simulink model "headway_sim"  (R2020a)
settings: Solver=VariableStepAuto  StartTime=0.0  StopTime=800  RelTol=1e-3
values from neighbouring files (symbols this model uses):
  A = eval(A)    [headway.m]
  B = eval(B)    [headway.m]
  Cd = 1.2    [headway.m]
  i_e = 100    [headway.m]
  id1_ref = 0    [headway.m]
  id2_ref = 0    [headway.m]
  iq1_ref = (Fx1_ref)/((3/2)*(pi/tau)*(Ld*(M/Ld)*i_e))    (= 482.136730936)    [headway.m]
  iq2_ref = (Fx2_ref)/((3/2)*(pi/tau)*(Ld*(M/Ld)*i_e))    (= 482.136730936)    [headway.m]
  Ld = 0.06    [headway.m]
  Lq = 0.06    [headway.m]
  M = 0.1    [headway.m]
  m = 60000    [headway.m]
  p = 3    [headway.m]
  R = 1.04    [headway.m]
  rho = 1.225    [headway.m]
  Sa = 13    [headway.m]
  tau = 1    [headway.m]
  Vref = [Vq1_ref;Vd1_ref;Vq2_ref;Vd2_ref]    [headway.m]
  x_ref = [iq1_ref; id1_ref; iq2_ref; id2_ref; xdot_ref]    [headway.m]
undefined symbols (not defined in the file or in its folder): K
settings Model: Creator=adelina  LastModifiedBy=Federico

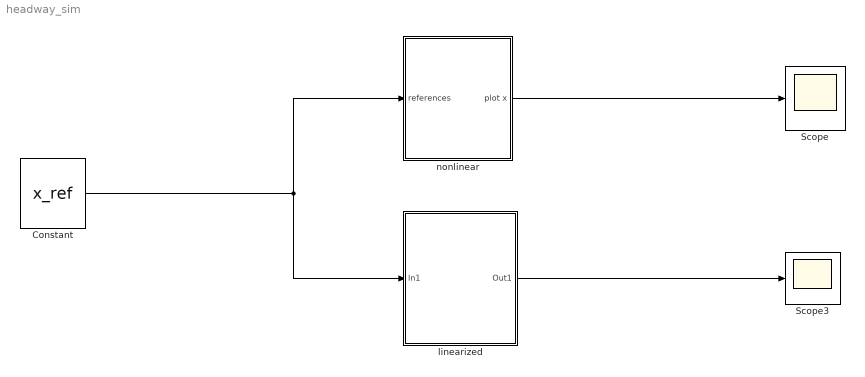
== system headway_sim ==
  Constant : Constant  Value=x_ref
  Scope : Scope
  Scope3 : Scope
  linearized : Subsystem
  nonlinear : Subsystem
  wires:
  Constant/1 -> nonlinear/1(references), linearized/1(In1)
  linearized/1(Out1) -> Scope3/1
  nonlinear/1(plot x) -> Scope/1

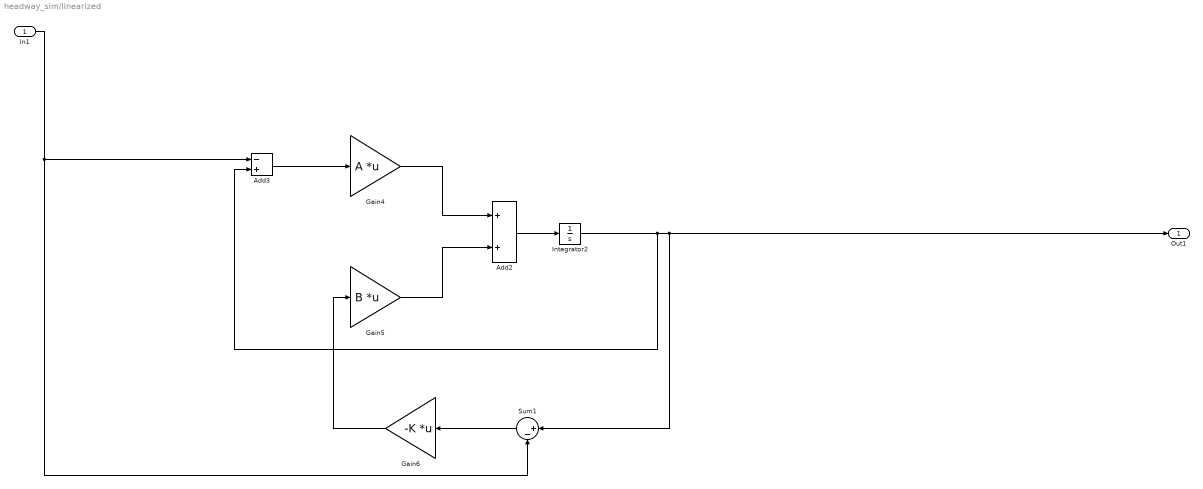
== system headway_sim/linearized ==
  In1 : Inport
  Add2 : Sum
  Add3 : Sum  Inputs=-+
  Gain4 : Gain  Gain=A  Multiplication=Matrix(K*u)
  Gain5 : Gain  Gain=B  Multiplication=Matrix(K*u)
  Gain6 : Gain  Gain=-K  Multiplication=Matrix(K*u)
  Integrator2 : Integrator  InitialCondition=[0;0;0;0;0]
  Sum1 : Sum  Inputs=|+-
  Out1 : Outport
  wires:
  Add2/1 -> Integrator2/1
  Gain5/1 -> Add2/2
  Gain6/1 -> Gain5/1
  Gain4/1 -> Add2/1
  Integrator2/1 -> Out1/1, Sum1/1, Add3/2
  Add3/1 -> Gain4/1
  In1/1 -> Sum1/2, Add3/1
  Sum1/1 -> Gain6/1

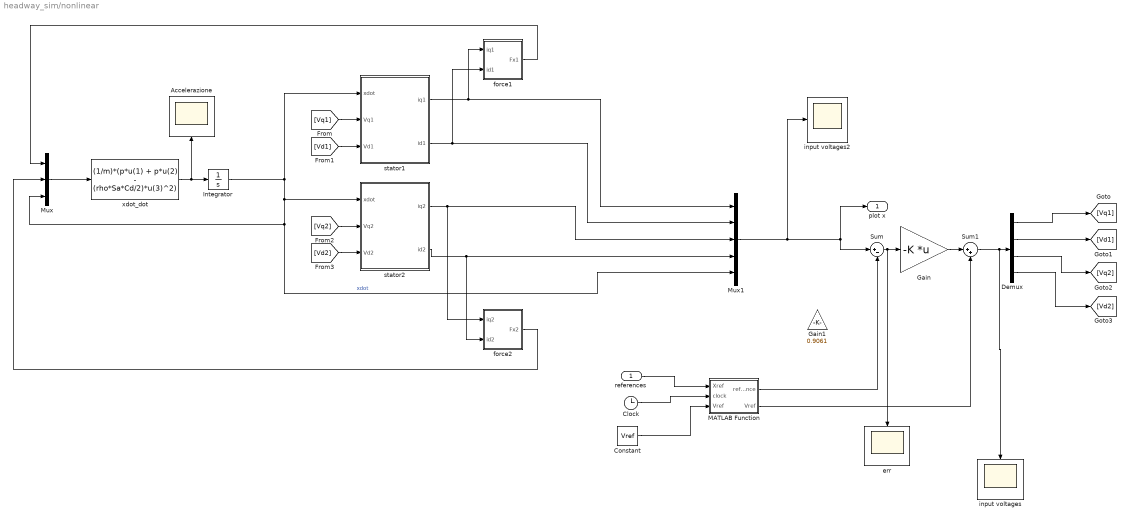
== system headway_sim/nonlinear ==
  references : Inport
  Accelerazione : Scope
  Clock : Clock
  Constant : Constant  Value=Vref
  Demux : Demux
  Gain : Gain  Gain=-K  Multiplication=Matrix(K*u)
  Gain1 : Gain  Gain=0.9061
  Integrator : Integrator
  MATLAB Function : MATLAB Function  TreatAsAtomicUnit=on
  Mux : Mux  Inputs=3
  Mux1 : Mux  Inputs=5
  Sum : Sum  Inputs=|+-
  Sum1 : Sum  Inputs=|++
  err : Scope
  force1 : Subsystem
  force2 : Subsystem
  input voltages : Scope
  input voltages2 : Scope
  stator1 : Subsystem
  stator2 : Subsystem
  xdot_dot : Fcn  Expr=(1/m)*(p*u(1) + p*u(2) - (rho*Sa*Cd/2)*u(3)^2)
  plot x : Outport
  wires:
  stator1/2(id1) -> Mux1/2, force1/2(id1)
  Mux1/1 -> input voltages2/1, Sum/1, plot x/1
  force1/1(Fx1) -> Mux/1
  Integrator/1 -> Mux/3, Mux1/5, stator2/1(xdot), stator1/1(xdot)  "xdot"
  Sum/1 -> Gain/1, err/1
  force2/1(Fx2) -> Mux/2
  stator2/1(iq2) -> force2/1("iq2 "), Mux1/3
  Mux/1 -> xdot_dot/1
  xdot_dot/1 -> Integrator/1, Accelerazione/1
  stator1/1(iq1) -> Mux1/1, force1/1("iq1 ")
  Demux/1 -> [Vq1]
  Demux/2 -> [Vd1]
  Demux/3 -> [Vq2]
  Demux/4 -> [Vd2]
  [Vq1] -> stator1/2(Vq1)
  [Vd1] -> stator1/3(Vd1)
  [Vq2] -> stator2/2(Vq2)
  [Vd2] -> stator2/3(Vd2)
  stator2/2(id2) -> force2/2(id2), Mux1/4
  Clock/1 -> MATLAB Function/2(clock)
  references/1 -> MATLAB Function/1(Xref)
  MATLAB Function/1(reference) -> Sum/2
  Gain/1 -> Sum1/1
  Sum1/1 -> input voltages/1, Demux/1
  MATLAB Function/2(Vref) -> Sum1/2
  Constant/1 -> MATLAB Function/3("Vref ")

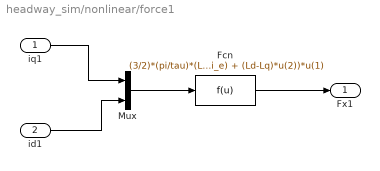
== system headway_sim/nonlinear/force1 ==
  "iq1 " : Inport
  id1 : Inport  Port=2
  Fcn : Fcn  Expr=(3/2)*(pi/tau)*(Ld*((M/Ld)*i_e) + (Ld-Lq)*u(2))*u(1)
  Mux : Mux  Inputs=2
  Fx1 : Outport
  wires:
  Fcn/1 -> Fx1/1
  "iq1 "/1 -> Mux/1
  id1/1 -> Mux/2
  Mux/1 -> Fcn/1

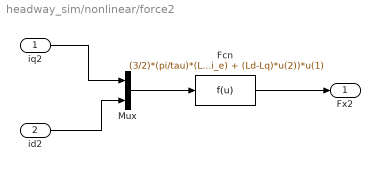
== system headway_sim/nonlinear/force2 ==
  "iq2 " : Inport
  id2 : Inport  Port=2
  Fcn : Fcn  Expr=(3/2)*(pi/tau)*(Ld*((M/Ld)*i_e) + (Ld-Lq)*u(2))*u(1)
  Mux : Mux  Inputs=2
  Fx2 : Outport
  wires:
  Fcn/1 -> Fx2/1
  "iq2 "/1 -> Mux/1
  id2/1 -> Mux/2
  Mux/1 -> Fcn/1

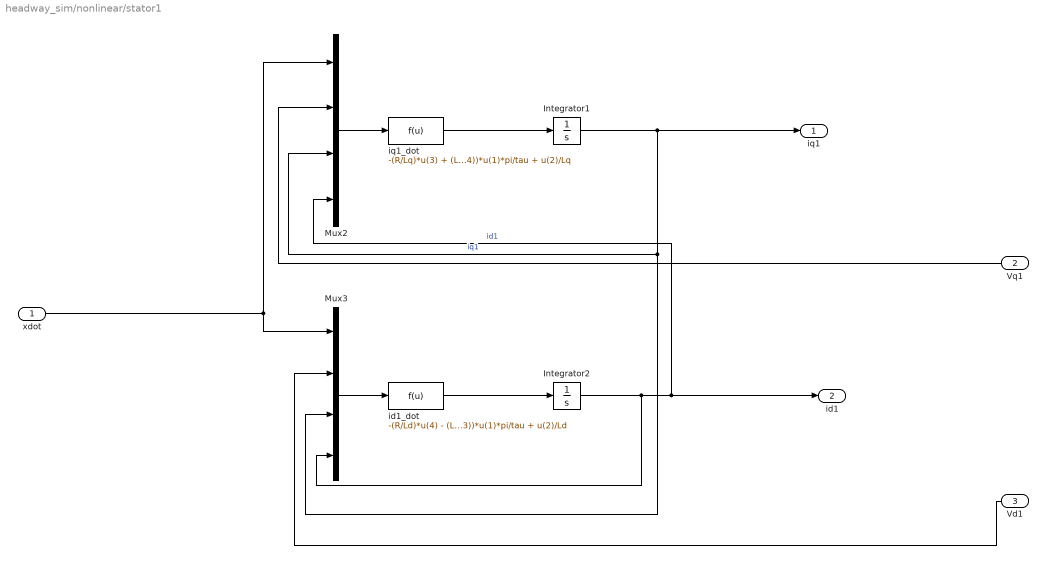
== system headway_sim/nonlinear/stator1 ==
  xdot : Inport
  Vq1 : Inport  Port=2
  Vd1 : Inport  Port=3
  Integrator1 : Integrator  InitialCondition=iq1_ref
  Integrator2 : Integrator  InitialCondition=id1_ref
  Mux2 : Mux
  Mux3 : Mux
  id1_dot : Fcn  Expr=-(R/Ld)*u(4) - (Lq/Ld)*(u(3))*u(1)*pi/tau + u(2)/Ld
  iq1_dot : Fcn  Expr=-(R/Lq)*u(3) + (Ld/Lq)*((M/Ld)*i_e + u(4))*u(1)*pi/tau + u(2)/Lq
  iq1 : Outport
  id1 : Outport  Port=2
  wires:
  iq1_dot/1 -> Integrator1/1
  Mux3/1 -> id1_dot/1
  Mux2/1 -> iq1_dot/1
  Vd1/1 -> Mux3/2
  id1_dot/1 -> Integrator2/1
  xdot/1 -> Mux2/1, Mux3/1
  Integrator1/1 -> Mux2/3, Mux3/3, iq1/1  "iq1"
  Integrator2/1 -> Mux3/4, Mux2/4, id1/1  "id1"
  Vq1/1 -> Mux2/2

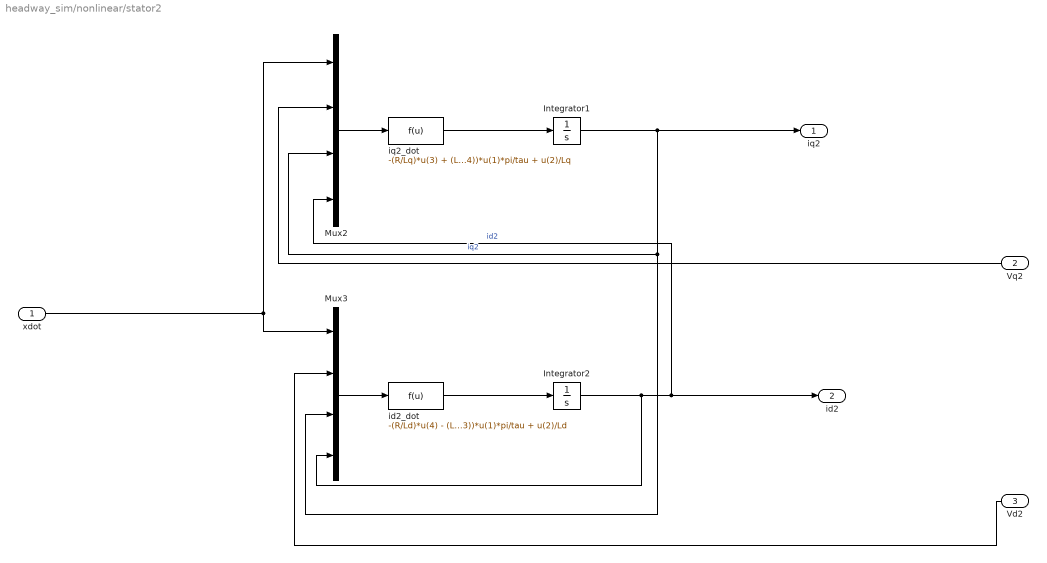
== system headway_sim/nonlinear/stator2 ==
  xdot : Inport
  Vq2 : Inport  Port=2
  Vd2 : Inport  Port=3
  Integrator1 : Integrator  InitialCondition=iq2_ref
  Integrator2 : Integrator  InitialCondition=id2_ref
  Mux2 : Mux
  Mux3 : Mux
  id2_dot : Fcn  Expr=-(R/Ld)*u(4) - (Lq/Ld)*(u(3))*u(1)*pi/tau + u(2)/Ld
  iq2_dot : Fcn  Expr=-(R/Lq)*u(3) + (Ld/Lq)*((M/Ld)*i_e + u(4))*u(1)*pi/tau + u(2)/Lq
  iq2 : Outport
  id2 : Outport  Port=2
  wires:
  iq2_dot/1 -> Integrator1/1
  Mux3/1 -> id2_dot/1
  Mux2/1 -> iq2_dot/1
  Vd2/1 -> Mux3/2
  id2_dot/1 -> Integrator2/1
  xdot/1 -> Mux2/1, Mux3/1
  Integrator1/1 -> Mux2/3, Mux3/3, iq2/1  "iq2"
  Integrator2/1 -> Mux3/4, Mux2/4, id2/1  "id2"
  Vq2/1 -> Mux2/2

== matlab function headway_sim/nonlinear/MATLAB Function ==
  data: Xref input; reference output; clock input; Vref output; Vref input
function [reference,Vref]= fcn(Xref,clock,Vref)
%% Solo Accelerazione
% steadyTime = 220; %più o meno come quello del paper mandato da luca. Comunque l'accelerazione sembra rimanere molto contenuta
% t = clock;
% 
% if t <= steadyTime
%     ramp = (1/steadyTime)*t;
% else
%     ramp = 1;
% end
% 
% % reference(5)=reference(5)*ramp; % Questo fa crescere sotto forma di rampa
% % solamente la velocità
% reference = Xref*ramp; %con questo tutte le grandezze crescono come una rampa nel tempo, tende a rendere leggermente più lento l'aumento della velocità ma non è troppo evidente

%% Accelerazione + decelerazione

%profilo trapezoidale per la velocità
%Ogni volta che si accelera decelera o altro viene introdotto un ritardo di
%x secondi. Questo ritardo dipende dal valore di i_e che nel nostro caso lavora come disturbo,
%se i_e=100 il ritardo è di circa 20 secondi quindi se voglio accelerare per 220 secondi setadyTime 
%dev'essere uguale a 200 e lo stesso vale per gli altri valori
steadyTime = 200; %più o meno come quello del paper mandato da luca. Comunque l'accelerazione sembra rimanere molto contenuta
crocera = 180; %secondi in cui il treno va a massima velocità
decelerazione = 180; % secondi necessari alla decelerazione del treno
t = clock; % tempo della simulazione


if t <= steadyTime
    ramp = (1/steadyTime)*t;
elseif and(t > steadyTime, t< steadyTime + crocera)
    ramp = 1;
elseif and(t >= steadyTime + crocera,t <= steadyTime + crocera + decelerazione)
    ramp = 1 - (1/decelerazione)*(t -(steadyTime + crocera));
else
    ramp = 0;
end

reference = Xref*ramp; %con questo tutte le grandezze crescono come una rampa nel tempo, tende a rendere leggermente più lento l'aumento della velocità ma non è troppo evidente

Vref=Vref*ramp;
